simulink model "s_qube2_rotpen_tf"  (R2013a)
settings: Solver=ode1  StartTime=0.0  StopTime=20  FixedStep=0.002  RelTol=1e-3
undefined symbols (not defined in the file or in its folder): arm_den, arm_num, pen_den, pen_num
libraries: simulink_extras x3
settings Model: ExtModeTrigDuration=5000  Creator=MLevis  LastModifiedBy=MLevis
settings SolverCC: PositivePriorityOrder=on
settings OptimizationCC: ExpressionDepthLimit=2147483647
settings RTWCC: SystemTargetFile=quarc_win64.tlc  TemplateMakefile=quarc_default_tmf  Description=QUARC Win64 Target  ProcessScript=quarc_win64_make_rtw_hook
settings STFCustomTargetCC: TargetPreCompLibLocation=C:\PROGRA~3\QUARC\lib\2013a\win64\release  GeneratePreprocessorConditionals=Disable all  CombineOutputUpdateFcns=on  SystemTargetFile=quarc_win64.tlc
settings GRTTargetCC: TargetPreCompLibLocation=C:\PROGRA~3\QUARC\lib\2013a\win64\release  ParMdlRefBuildCompliant=off  CompOptLevelCompliant=off  ConcurrentExecutionCompliant=off  MatFileLogging=off  ExtMode=on  ExtModeMexFile=quarc_comm

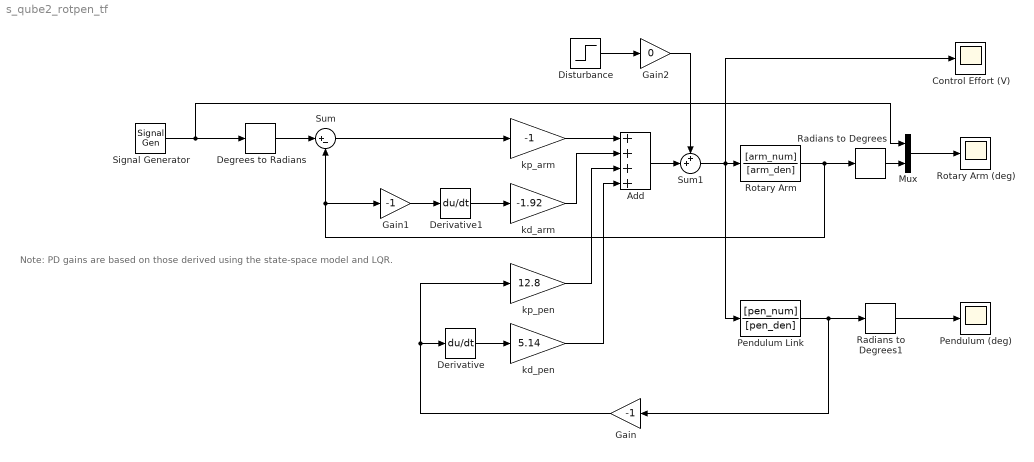
== system s_qube2_rotpen_tf ==
  note: Note: PD gains are based on those derived
      | using the state-space model and LQR.
  Add : Sum  Inputs=++++
  Control Effort (V) : Scope
      settings: TimeRange=20  YMin=-10  YMax=10  SaveName=ScopeData2  MaxDataPoints=10000
  Degrees to Radians : simulink_extras/Transformations/Degrees to Radians
  Derivative : Derivative
  Derivative1 : Derivative
  Disturbance : Step  SampleTime=0
  Gain : Gain  Gain=-1
  Gain1 : Gain  Gain=-1
  Gain2 : Gain  Gain=0
  Mux : Mux  Inputs=2
  Pendulum (deg) : Scope
      settings: TimeRange=20  YMin=-20  YMax=20  MaxDataPoints=10000
  Pendulum Link : TransferFcn  Numerator=[pen_num]  Denominator=[pen_den]
  Radians to Degrees : simulink_extras/Transformations/Radians to Degrees
  Radians to Degrees1 : simulink_extras/Transformations/Radians to Degrees
  Rotary Arm : TransferFcn  Numerator=[arm_num]  Denominator=[arm_den]
  Rotary Arm (deg) : Scope
      settings: TimeRange=20  YMin=-75  YMax=75  MaxDataPoints=10000
  Signal Generator : SignalGenerator  WaveForm=square  Amplitude=30  Frequency=0.08
  Sum : Sum  Inputs=|+-
  Sum1 : Sum  Inputs=++|
  kd_arm : Gain  Gain=-1.92
  kd_pen : Gain  Gain=5.14
  kp_arm : Gain  Gain=-1
  kp_pen : Gain  Gain=12.8
  wires:
  Sum/1 -> kp_arm/1
  kp_arm/1 -> Add/1
  Derivative/1 -> kd_pen/1
  Rotary Arm/1 -> Gain1/1, Sum/2, Radians to Degrees/1
  Derivative1/1 -> kd_arm/1
  Mux/1 -> Rotary Arm (deg)/1
  Degrees to Radians/1 -> Sum/1
  Radians to Degrees/1 -> Mux/2
  Radians to Degrees1/1 -> Pendulum (deg)/1
  kd_arm/1 -> Add/2
  kp_pen/1 -> Add/3
  kd_pen/1 -> Add/4
  Gain/1 -> kp_pen/1, Derivative/1
  Gain1/1 -> Derivative1/1
  Pendulum Link/1 -> Radians to Degrees1/1, Gain/1
  Sum1/1 -> Control Effort (V)/1, Pendulum Link/1, Rotary Arm/1
  Add/1 -> Sum1/2
  Disturbance/1 -> Gain2/1
  Gain2/1 -> Sum1/1
  Signal Generator/1 -> Mux/1, Degrees to Radians/1
